simulink model "Experiment2_PID_model"  (R2018b)
settings: Solver=ode1  StartTime=0.0  StopTime=simulink_time  FixedStep=step_size  RelTol=1e-3  EnableMultiTasking=on
values from neighbouring files (symbols this model uses):
  exp_model = 0    [model_ref.mat]
  Kd1 = 0.1    [ref1.mat]
  Ki1 = 0.25    [ref1.mat]
  Kp1 = 1    [ref1.mat]
  Plant_K = 174.56    [Student_ref.mat]
  Plant_T1 = 0.07124    [Student_ref.mat]
undefined symbols (not defined in the file or in its folder): Plant_T2, simulink_start_time
libraries: simulink x1
settings Model: Creator=Administrator  LastModifiedBy=QJ-
settings DataIOCC: LimitDataPoints=on  SaveFormat=Array
settings OptimizationCC: ExpressionDepthLimit=2147483647  LifeSpan=inf
settings DebuggingCC: UnderspecifiedInitializationDetection=Classic  MergeDetectMultiDrivingBlocksExec=none  SolverPrmCheckMsg=warning  StateNameClashWarn=warning  SFUnexpectedBacktrackingDiag=warning  SFNoUnconditionalDefaultTransitionDiag=warning  SFExecutionAtInitializationDiag=none
settings HardwareCC: ProdBitPerPointer=32  ProdBitPerSizeT=32  ProdBitPerPtrDiffT=32  ProdLargestAtomicFloat=None  ProdIntDivRoundTo=Undefined  ProdEndianess=Unspecified  ProdWordSize=32  ProdHWDeviceType=32-bit Generic
settings ModelReferenceCC: PropagateSignalLabelsOutOfModel=off
settings SFSimCC: SimUseLocalCustomCode=off
settings RTWCC: RTWUseLocalCustomCode=off
settings CodeAppCC: StateflowObjectComments=on
settings GRTTargetCC: TargetLangStandard=C89/C90 (ANSI)  GeneratePreprocessorConditionals=Disable all
settings ConfigComp: CovMetricSettings=dw  CovHtmlReporting=on  CovSaveCumulativeToWorkspaceVar=on  CovSaveSingleToWorkspaceVar=on  CovExternalEMLEnable=off

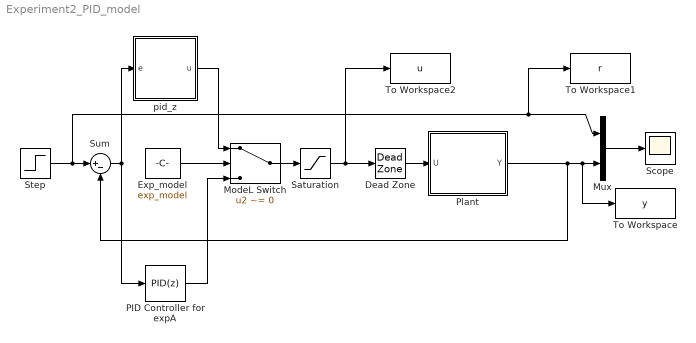
== system Experiment2_PID_model ==
  Dead Zone : DeadZone  LowerValue=-2  UpperValue=2  SaturateOnIntegerOverflow=on
  Exp_model : Constant  Value=exp_model
  ModeL Switch : Switch  Criteria=u2 ~= 0
  Mux : Mux  Inputs=2
  PID Controller for expA : simulink/Continuous/PID Controller  Controller=PID  Form=Parallel  TimeDomain=Discrete-time  SampleTime=0.002  IntegratorMethod=Trapezoidal  FilterMethod=Trapezoidal  ControllerParametersSource=internal  P=Kp1  I=Ki1  D=Kd1  UseFilter=off  N=100  TunerSelectOption=Transfer Function Based (PID Tuner App)  InitialConditionSource=internal  InitialConditionForIntegrator=0  InitialConditionForFilter=0  DifferentiatorICPrevScaledInput=0  ExternalReset=none  TrackingMode=off  Kt=1  LimitOutput=off  UpperSaturationLimit=inf  LowerSaturationLimit=-inf  LinearizeAsGain=on  AntiWindupMode=none  Kb=1  POutMin=[]  POutMax=[]  IOutMin=[]  IOutMax=[]  DOutMin=[]  DOutMax=[]  NOutMin=[]  NOutMax=[]  SumOutMin=[]  SumOutMax=[]  SaturationOutMin=[]  SaturationOutMax=[]  PParamMin=[]  PParamMax=[]  IParamMin=[]  IParamMax=[]  DParamMin=[]  DParamMax=[]  NParamMin=[]  NParamMax=[]  KbParamMin=[]  KbParamMax=[]  KtParamMin=[]  KtParamMax=[]  KbOutMin=[]  KbOutMax=[]  KtOutMin=[]  KtOutMax=[]  IntegratorOutMin=[]  IntegratorOutMax=[]  FilterOutMin=[]  FilterOutMax=[]  SumI1OutMin=[]  SumI1OutMax=[]  SumI2OutMin=[]  SumI2OutMax=[]  SumI3OutMin=[]  SumI3OutMax=[]  SumI4OutMin=[]  SumI4OutMax=[]  SumDOutMin=[]  SumDOutMax=[]  DifferentiatorOutMin=[]  DifferentiatorOutMax=[]  FilterDiffOutCoefMin=[]  FilterDiffOutCoefMax=[]  ReciprocalOutMin=[]  ReciprocalOutMax=[]  SumDenOutMin=[]  SumDenOutMax=[]  SumNumOutMin=[]  SumNumOutMax=[]  DivideOutMin=[]  DivideOutMax=[]  IntegratorContinuousStateAttributes=''  IntegratorStateMustResolveToSignalObject=off  IntegratorRTWStateStorageClass=Auto  FilterContinuousStateAttributes=''  FilterStateMustResolveToSignalObject=off  FilterRTWStateStorageClass=Auto  ParallelPVariant=InternalParameters  IdealPVariant=Disabled  IVariant=InternalParameters  DVariant=InternalParameters  IntegratorVariant=Discrete  SatVariant=Disabled  AWVariant=Passthrough  PCopyVariant=Disabled  TRVariant=Disabled  FdbkBlocksVariant=Forward  IdealPFdbkVariant=Disabled  SatFdbkVariant=Disabled  DerivativeFilterVariant=Differentiator  NVariant=Passthrough  NCopyVariant=Disabled_SignalSpec  FilterICVariant=InternalICsDifferentiator  IntegratorICVariant=InternalICs  ExternalResetVariant=Disabled  TRSumVariant=Passthrough  SumFdbkVariant=Disabled  SumVariant=Sum_PID
  Plant : Subsystem
  Saturation : Saturate  UpperLimit=19.2  LowerLimit=-19.2
  Scope : Scope
  Step : Step  Time=simulink_start_time  After=60  SampleTime=0
  Sum : Sum  Inputs=|+-
  To Workspace : ToWorkspace  VariableName=y  SampleTime=-1
  To Workspace1 : ToWorkspace  VariableName=r  SampleTime=-1
  To Workspace2 : ToWorkspace  VariableName=u  SampleTime=-1
  pid_z : Subsystem
  wires:
  Step/1 -> To Workspace1/1, Mux/1, Sum/1
  Mux/1 -> Scope/1
  ModeL Switch/1 -> Saturation/1
  Saturation/1 -> To Workspace2/1, Dead Zone/1
  Plant/1(Y) -> To Workspace/1, Mux/2, Sum/2
  Dead Zone/1 -> Plant/1(U)
  Exp_model/1 -> ModeL Switch/2
  Sum/1 -> PID Controller for expA/1, pid_z/1(e)
  pid_z/1(u) -> ModeL Switch/1
  PID Controller for expA/1 -> ModeL Switch/3

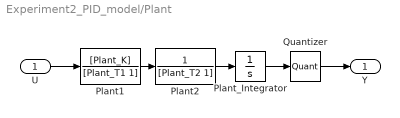
== system Experiment2_PID_model/Plant ==
  U : Inport
  Plant1 : TransferFcn  Numerator=[Plant_K]  Denominator=[Plant_T1 1]
  Plant2 : TransferFcn  Denominator=[Plant_T2 1]
  Plant_Integrator : Integrator
  Quantizer : Quantizer  QuantizationInterval=0.01
  Y : Outport
  wires:
  U/1 -> Plant1/1
  Quantizer/1 -> Y/1
  Plant1/1 -> Plant2/1
  Plant_Integrator/1 -> Quantizer/1
  Plant2/1 -> Plant_Integrator/1

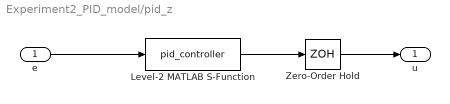
== system Experiment2_PID_model/pid_z ==
  e : Inport
  Level-2 MATLAB S-Function : M-S-Function  FunctionName=pid_controller  Parameters=Kp1, Ki1, Kd1
  Zero-Order Hold : ZeroOrderHold  SampleTime=-1
  u : Outport
  wires:
  e/1 -> Level-2 MATLAB S-Function/1
  Zero-Order Hold/1 -> u/1
  Level-2 MATLAB S-Function/1 -> Zero-Order Hold/1
